simulink model "stim_remover"  (R2014a)
settings: Solver=ode45  StartTime=0.0  StopTime=10.0  RelTol=1e-3
settings Model: Creator=BETHEL.OSUAGWU  LastModifiedBy=BETHEL.OSUAGWU

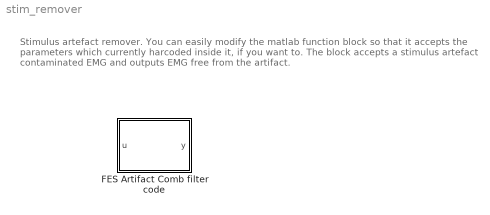
== system stim_remover ==
  note: Stimulus artefact remover.
      | You can easily modify the matlab function block so that it accepts
      | the parameters which currently harcoded inside it, if you want to.
      |
      | The block accepts a stimulus artefact contaminated EMG and outputs EMG free from the artifact.
  FES Artifact Comb filter code : MATLAB Function  TreatAsAtomicUnit=on

== matlab function stim_remover/FES Artifact Comb filter code ==
  data: u input; y output
function y  = fcn(u)
%#codegen

persistent u_mem;
fes_freq=25;%FES frequency
Fs=1000;%EMG/data samplerate
K=40;%round(Fs/fes_freq); %Comb filter order = (1/fes_freq)*Fs
a=-1;%{-1 to 0}
if isempty(u_mem)
    u_mem=zeros(K,1);
end





%% Comb filtering
% Forward comb
y=u+ a*u_mem(1);



u_mem(1:end-1)=u_mem(2:end);
u_mem(end)=u;



end





%
